simulink model "actuatorKalman"  (R2025b)
settings: Solver=FixedStepDiscrete  StartTime=0.0  StopTime=10.0  RelTol=1e-3
settings Model: Creator=karadeli  LastModifiedBy=karadeli
settings OptimizationCC: DefaultParameterBehavior=Inlined  UseDivisionForNetSlopeComputation=on  GainParamInheritBuiltInType=on  UseFloatMulNetSlope=on  InlineInvariantSignals=on  PassReuseOutputArgsAs=Individual arguments  ZeroExternalMemoryAtStartup=off  ZeroInternalMemoryAtStartup=off  NoFixptDivByZeroProtection=on  EfficientFloat2IntCast=on  LifeSpan=1  OptimizeBlockOrder=speed  DifferentSizesBufferReuse=on  EfficientTunableParamExpr=on
settings DebuggingCC: ParameterTunabilityLossMsg=error
settings HardwareCC: ProdBitPerPointer=32.0  ProdBitPerSizeT=32.0  ProdBitPerPtrDiffT=32.0  ProdLargestAtomicInteger=Long  ProdLargestAtomicFloat=Double  ProdWordSize=32.0  ProdLongLongMode=on  ProdHWDeviceType=ARM Compatible->ARM Cortex-M  TargetBitPerInt=16.0  TargetBitPerPointer=16.0  TargetBitPerSizeT=16.0  TargetBitPerPtrDiffT=16.0  TargetLongLongMode=on  TargetIntDivRoundTo=Zero  TargetEndianess=LittleEndian  TargetWordSize=16.0  TargetHWDeviceType=STMicroelectronics->ST10/Super10
settings SFSimCC: MATLABDynamicMemAlloc=off
settings RTWCC: SystemTargetFile=ert.tlc  GenCodeOnly=on  TemplateMakefile=ert_default_tmf  TargetLang=C++  GenerateCodeMetricsReport=on  Description=Embedded Coder
settings CodeAppCC: ForceParamTrailComments=on  IgnoreCustomStorageClasses=off  OperatorAnnotations=on  SimulinkDataObjDesc=on  SFDataObjDesc=on  CustomSymbolStrGlobalVar=rt$N$M  CustomSymbolStrType=$N$M  CustomSymbolStrFcn=$N$M$F  CustomSymbolStrMacro=$N$M  InsertBlockDesc=on
settings ERTTargetCC: RootIOFormat=Structure reference  ERTCustomFileTemplate=example_file_process.tlc  ERTFilePackagingFormat=CompactWithDataFile  TargetLangStandard=C++11 (ISO)  GenerateSampleERTMain=on  IncludeMdlTerminateFcn=off  CombineSignalStateStructs=on  SupportAbsoluteTime=off  CodeInterfacePackaging=C++ class  SubcomponentCodeInterfacePackaging=C++ class  SupportComplex=off  SupportNonInlinedSFcns=on  RemoveDisableFunc=on

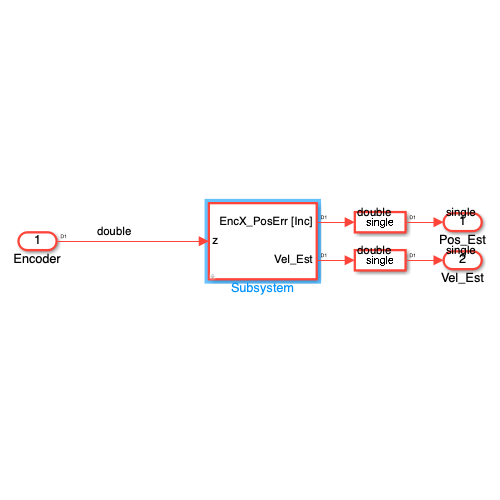
[thumbnail: Simulink's stored preview of the top-level diagram]
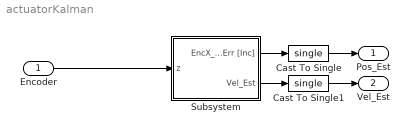
== system actuatorKalman ==
  Encoder : Inport  PortDimensions=1  SampleTime=1/4000
  Cast To Single : DataTypeConversion  OutDataTypeStr=single  SaturateOnIntegerOverflow=off  RndMeth=Floor
  Cast To Single1 : DataTypeConversion  OutDataTypeStr=single  SaturateOnIntegerOverflow=off  RndMeth=Floor
  Subsystem : Subsystem  mask{Ts=1/4000, lambda_RQ=0.01}
  Pos_Est : Outport
  Vel_Est : Outport  Port=2
  wires:
  Subsystem/1(EncX_PosErr [Inc]) -> Cast To Single/1
  Subsystem/2(Vel_Est) -> Cast To Single1/1
  Encoder/1 -> Subsystem/1(z)
  Cast To Single/1 -> Pos_Est/1
  Cast To Single1/1 -> Vel_Est/1

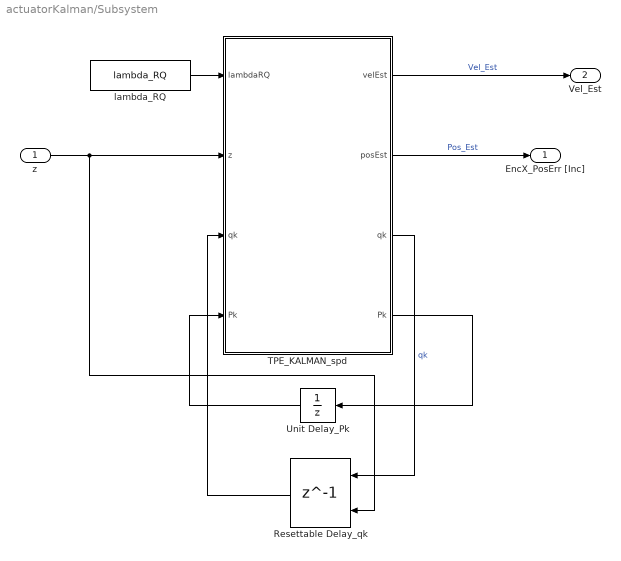
== system actuatorKalman/Subsystem ==
  z : Inport  Unit=deg  PortDimensions=1
  Resettable Delay_qk : Delay  DelayLength=1  InitialConditionSource=Input port  SampleTime=Ts
      settings: InputPortMap=u0,p4
  TPE_KALMAN_spd : MATLAB Function  TreatAsAtomicUnit=on
  Unit Delay_Pk : UnitDelay  InitialCondition=[0.155 65; 65 5.7e4]  SampleTime=Ts  HasFrameUpgradeWarning=on
  lambda_RQ : Constant  Value=lambda_RQ  OutDataTypeStr=double
  EncX_PosErr [Inc] : Outport  OutDataTypeStr=double  Unit=deg  PortDimensions=1  SampleTime=Ts  VectorParamsAs1DForOutWhenUnconnected=off
  Vel_Est : Outport  Port=2  OutDataTypeStr=double  Unit=deg/s  PortDimensions=1  SampleTime=Ts  VectorParamsAs1DForOutWhenUnconnected=off
  wires:
  Resettable Delay_qk/1 -> TPE_KALMAN_spd/3("qk ")
  Unit Delay_Pk/1 -> TPE_KALMAN_spd/4("Pk ")
  lambda_RQ/1 -> TPE_KALMAN_spd/1(lambdaRQ)
  TPE_KALMAN_spd/3(qk) -> Resettable Delay_qk/1  "qk"
  z/1 -> TPE_KALMAN_spd/2(z), Resettable Delay_qk/2
  TPE_KALMAN_spd/1(velEst) -> Vel_Est/1  "Vel_Est"
  TPE_KALMAN_spd/2(posEst) -> EncX_PosErr [Inc]/1  "Pos_Est"
  TPE_KALMAN_spd/4(Pk) -> Unit Delay_Pk/1

== matlab function actuatorKalman/Subsystem/TPE_KALMAN_spd ==
  settings: updateMethod=DISCRETE  sampleTime=Ts
  data z settings: description=since it reads the encoder data its made uint32
  data: lambdaRQ input double size=1; velEst output double size=1; posEst output double size=1; qk output size=[2,1]; z input double size=1; qk input double size=[2,1]; Pk input double size=[2,2]; Ts parameter double size=1; Pk output size=[2,2]
function [ velEst, posEst, qk,Pk] =Kalman_X_Enc(lambdaRQ,z, qk, Pk, Ts)
%   200814 
%   --------
% INPUTS
%  z: measurement (1,1) %    [increment]
%   q1: previous state [2Nx1]
%   P1: previous error cov matrix [2Nx2N]
%   qk1: previous state [2x1]
%   Pk1: previous error cov matrix [2x2]
%   nSpindle : Spindle Speed [rpm]
%   IncrSec: increment per second
% PARAMETERS Periodic component
%   Ts      : Sampling time [ms]
%   Q :  process noise covariance matrix [2x2], tunable
%   R  :  measurement noise cov 1x1, tunable

%   R olcerdeki hataa,
%   Q modeldeki hata, Q kuculurse modele guvenir, smooth olur. Ama aynı isi
%   disaridan lambdaRQ carpani ile yapabilirsin.
R_Enc=(360/65536)^2;
Q_Enc=[Ts^3/3, Ts^2/2; Ts^2/2, Ts]*(4/Ts)^2*1e-3;% <<<<<< BUNLA OYNA 1-4-10

%%  Remove the trend with kinematic Kalman Filter
Q=lambdaRQ*Q_Enc;
[qk,Pk] = Kalman_Kinematic(z, qk, Pk, R_Enc,Q,Ts);
velEst = qk(2);%[incr/sec]
posEst=qk(1);


end



function [q,P] = Kalman_Kinematic(z, q, P, R,Q,Ts)
%   First Eqn : Priori state est
PosPrior = q(1)+q(2)*Ts;
VelPrior =q(2);
%   Second Eqn : Priori cov matrix
dummy = P(2,1)+Ts*P(2,2);
P11 = P(1,1)+Ts*P(1,2) + Ts*dummy +Q(1,1);
P21 = dummy+Q(2,1);
P12 = P(1,2)+Ts*P(2,2)+Q(1,2);
P22 = P(2,2)+Q(2,2);

%   Kalman Gain
dummy = 1/(P11+R);
K1= P11*dummy;
K2= P21*dummy; % No need since there is no vel estimate

% State estimate
dummy=z-PosPrior;
q = [PosPrior + K1*dummy;...
    VelPrior+K2*dummy];

%   Covariance Matrix
P=[P11-K1*P11, P12-K1*P12;...
    P21-K2*P11, P22-K2*P12];
end
